simulink model "simulink_afbs_demo"  (R2015a)
settings: Solver=ode45  StartTime=0.0  StopTime=5  FixedStep=0.1  RelTol=1e-4
values from neighbouring files (symbols this model uses):
  sys = tf(sys_zpk)    [demo.m]
  T1 = 1000    [demo.m]
  T2 = 1000    [demo.m]
  T3 = 1000    [demo.m]
settings Model: Creator=Xiaotian  LastModifiedBy=Xiaotian

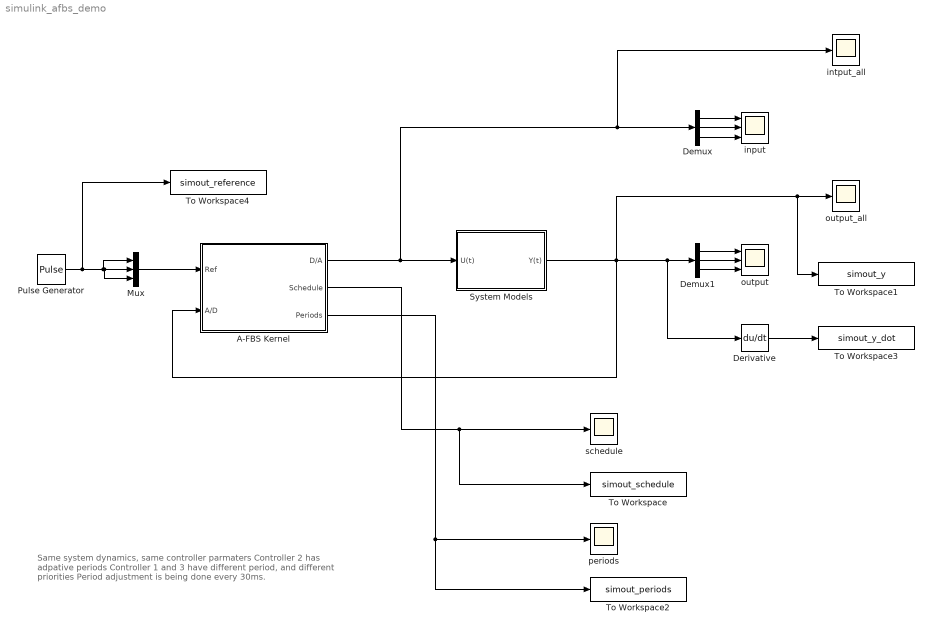
== system simulink_afbs_demo ==
  note: Same system dynamics, same controller parmaters
      | Controller 2 has adpative periods
      | Controller 1 and 3 have different period, and different priorities
      | Period adjustment is being done every 30ms.
  A-FBS Kernel : Subsystem
  Demux : Demux  Outputs=3
  Demux1 : Demux  Outputs=3
  Derivative : Derivative
  Mux : Mux  Inputs=3
  Pulse Generator : DiscretePulseGenerator  PulseType=Time based  Period=0.2  PulseWidth=50
  System Models : Subsystem
  To Workspace : ToWorkspace  VariableName=simout_schedule  SaveFormat=Timeseries  SampleTime=-1
  To Workspace1 : ToWorkspace  VariableName=simout_y  SaveFormat=Timeseries  SampleTime=-1
  To Workspace2 : ToWorkspace  VariableName=simout_periods  SaveFormat=Timeseries  SampleTime=-1
  To Workspace3 : ToWorkspace  VariableName=simout_y_dot  SaveFormat=Timeseries  SampleTime=-1
  To Workspace4 : ToWorkspace  VariableName=simout_reference  SaveFormat=Timeseries  SampleTime=-1
  input : Scope  NumInputPorts=3
      settings: YMin=-5~-5~-5  YMax=5~5~5
  intput_all : Scope
      settings: SaveName=ScopeData4
  output : Scope  NumInputPorts=3
      settings: YMin=-5~-5~-5  YMax=5~5~5
  output_all : Scope
      settings: SaveName=ScopeData3
  periods : Scope
      settings: SaveName=ScopeData5
  schedule : Scope
      settings: SaveName=ScopeData2
  wires:
  A-FBS Kernel/1(D/A) -> intput_all/1, Demux/1, System Models/1(U(t))
  A-FBS Kernel/2(Schedule) -> To Workspace/1, schedule/1
  System Models/1(Y(t)) -> A-FBS Kernel/2(A/D), Derivative/1, Demux1/1, To Workspace1/1, output_all/1
  Demux1/3 -> output/3
  Demux1/2 -> output/2
  Demux1/1 -> output/1
  Demux/3 -> input/3
  Demux/2 -> input/2
  Demux/1 -> input/1
  A-FBS Kernel/3(Periods) -> To Workspace2/1, periods/1
  Derivative/1 -> To Workspace3/1
  Pulse Generator/1 -> To Workspace4/1, Mux/1, Mux/3, Mux/2
  Mux/1 -> A-FBS Kernel/1(Ref)

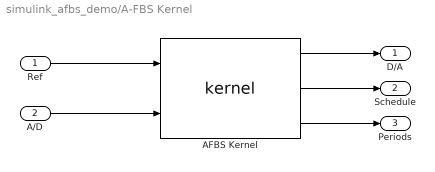
== system simulink_afbs_demo/A-FBS Kernel ==
  Ref : Inport
  A/D : Inport  Port=2
  AFBS Kernel : S-Function  FunctionName=kernel  Parameters=[T1, T2, T3]
  D/A : Outport
  Schedule : Outport  Port=2
  Periods : Outport  Port=3
  wires:
  AFBS Kernel/1 -> D/A/1
  AFBS Kernel/2 -> Schedule/1
  AFBS Kernel/3 -> Periods/1
  Ref/1 -> AFBS Kernel/1
  A/D/1 -> AFBS Kernel/2

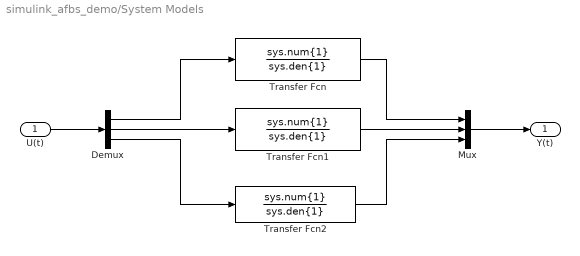
== system simulink_afbs_demo/System Models ==
  U(t) : Inport
  Demux : Demux  Outputs=3
  Mux : Mux  Inputs=3
  Transfer Fcn : TransferFcn  Numerator=sys.num{1}  Denominator=sys.den{1}
  Transfer Fcn1 : TransferFcn  Numerator=sys.num{1}  Denominator=sys.den{1}
  Transfer Fcn2 : TransferFcn  Numerator=sys.num{1}  Denominator=sys.den{1}
  Y(t) : Outport
  wires:
  U(t)/1 -> Demux/1
  Demux/1 -> Transfer Fcn/1
  Demux/2 -> Transfer Fcn1/1
  Demux/3 -> Transfer Fcn2/1
  Transfer Fcn/1 -> Mux/1
  Transfer Fcn1/1 -> Mux/2
  Transfer Fcn2/1 -> Mux/3
  Mux/1 -> Y(t)/1
